simulink model "no_connections"  (R2024b)
settings: Solver=VariableStepAuto  StartTime=0.0  StopTime=525  RelTol=1e-3
libraries: Solver_SF x1
settings Model: Creator=Pain  LastModifiedBy=Pain

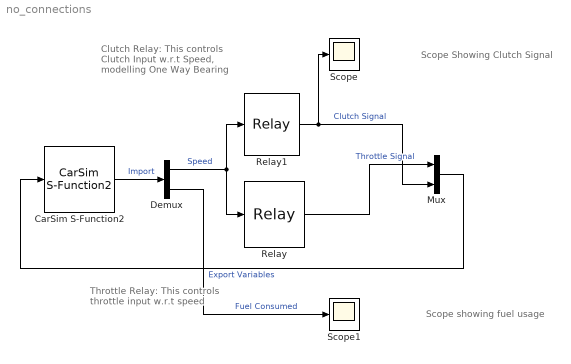
== system no_connections ==
  note: Scope Showing Clutch Signal
  note: Scope showing fuel usage
  note: Throttle Relay: This controls
      | throttle input w.r.t speed
  note: Clutch Relay: This controls Clutch
      | Input w.r.t Speed, modelling One Way
      | Bearing
  CarSim S-Function2 : Solver_SF/CarSim S-Function2  Priority=1  VehicleCode=i_i  SIMFILE=simfile.sim
      settings: AttributesFormatString=Vehicle Code: %<VehicleCode>  SourceProductName=CarSim S-Function
  Demux : Demux  Outputs=2
  Mux : Mux  Inputs=2
  Relay : Relay  OnSwitchValue=35.9  OffSwitchValue=15.5  OnOutputValue=0  OffOutputValue=0.3
  Relay1 : Relay  OnSwitchValue=35.9  OffSwitchValue=15
  Scope : Scope
  Scope1 : Scope
  wires:
  Relay/1 -> Mux/1  "Throttle Signal"
  Relay1/1 -> Mux/2, Scope/1  "Clutch Signal"
  Mux/1 -> CarSim S-Function2/1  "Export Variables"
  CarSim S-Function2/1 -> Demux/1  "Import"
  Demux/1 -> Relay/1, Relay1/1  "Speed"
  Demux/2 -> Scope1/1  "Fuel Consumed"
